simulink model "traction_circle"  (R2024b)
settings: Solver=FixedStepDiscrete  StartTime=t_0  StopTime=t_f  FixedStep=dt  RelTol=1e-5
undefined symbols (not defined in the file): final_side, final_slip, initial_side, initial_slip, t_0, t_f
libraries: simulink x2
settings Model: Creator=Yevgeniy Gorbachev  LastModifiedBy=yevge
settings SolverCC: ZeroCrossControl=DisableAll  ZeroCrossAlgorithm=Adaptive
settings DataIOCC: DatasetSignalFormat=timetable
settings RTWCC: GPUComputeCapability=3.5

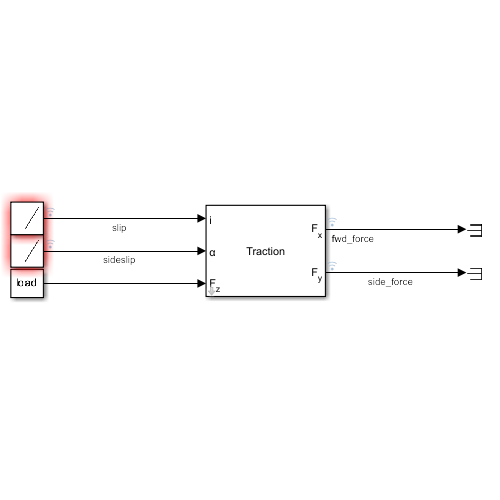
[thumbnail: Simulink's stored preview of the top-level diagram]
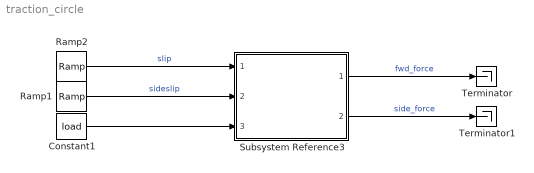
== system traction_circle ==
  Constant1 : Constant  Value=load
  Ramp1 : simulink/Sources/Ramp  slope=(final_side - initial_side) / (t_f - t_0)  start=t_0  InitialOutput=initial_side
  Ramp2 : simulink/Sources/Ramp  slope=(final_slip - initial_slip) / (t_f - t_0)  start=t_0  InitialOutput=initial_slip
  Subsystem Reference3 : Subsystem  ReferencedSubsystem=traction
  Terminator : Terminator
  Terminator1 : Terminator
  wires:
  Constant1/1 -> Subsystem Reference3/3
  Subsystem Reference3/2 -> Terminator1/1  "side_force"
  Subsystem Reference3/1 -> Terminator/1  "fwd_force"
  Ramp2/1 -> Subsystem Reference3/1  "slip"
  Ramp1/1 -> Subsystem Reference3/2  "sideslip"
